simulink model "Group_20"  (R2024b)
settings: Solver=VariableStepAuto  StartTime=0.0  StopTime=inf  RelTol=1e-3
undefined symbols (not defined in the file or in its folder): Ion, Lithium
libraries: spsBatteryLib x3, spsIdealSwitchLib x3, spsSeriesRLCLoadLib x3, spsVoltageMeasurementLib x1, sps_lib x1
settings Model: Creator=om  LastModifiedBy=om

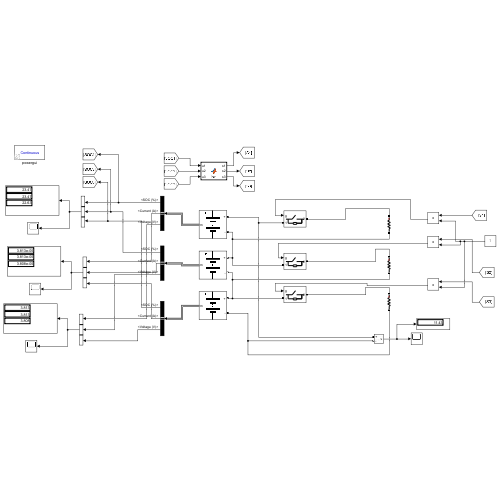
[thumbnail: Simulink's stored preview of the top-level diagram]
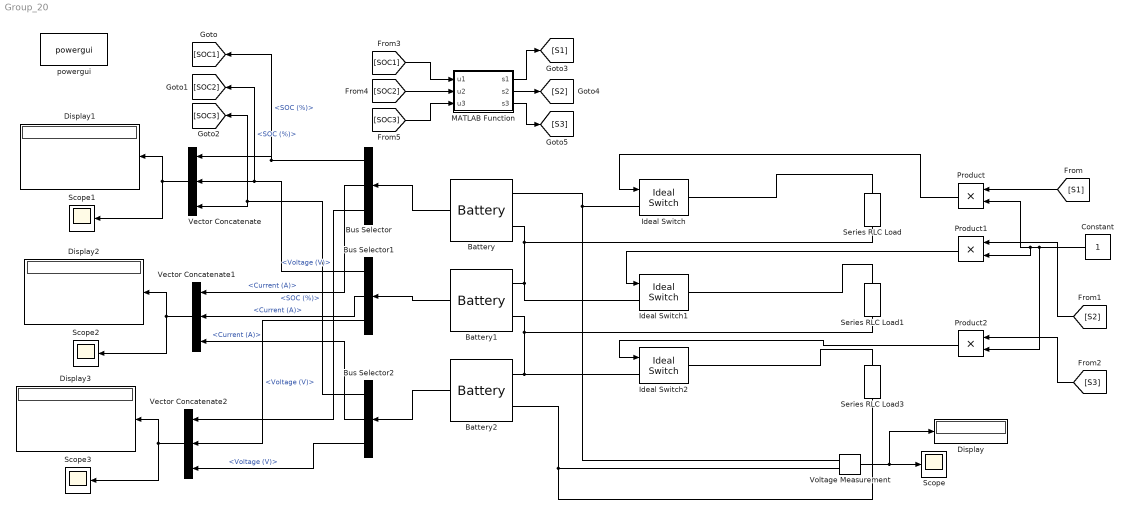
== system Group_20 ==
  Battery : spsBatteryLib/Battery  BatType=Lithium-Ion  NomV=3.6  NomQ=4.5  SOC=80  Batt_Tr=1  PresetModel=on  MaxQ=4.5  MinV=2.7  FullV=4.1904  Dis_rate=1.9565  R=0.008  Normal_OP=4.0696  expZone="[3.8894     0.22109]"
  Battery1 : spsBatteryLib/Battery  BatType=Lithium-Ion  NomV=3.6  NomQ=4.5  SOC=50  Batt_Tr=1  PresetModel=on  MaxQ=4.5  MinV=2.7  FullV=4.1904  Dis_rate=1.9565  R=0.008  Normal_OP=4.0696  expZone="[3.8894     0.22109]"
  Battery2 : spsBatteryLib/Battery  BatType=Lithium-Ion  NomV=3.6  NomQ=4.5  SOC=20  Batt_Tr=1  PresetModel=on  MaxQ=4.5  MinV=2.7  FullV=4.1904  Dis_rate=1.9565  R=0.008  Normal_OP=4.0696  expZone="[3.8894     0.22109]"
  Bus Selector : BusSelector  OutputSignals=SOC (%),Current (A),Voltage (V)
  Bus Selector1 : BusSelector  OutputSignals=SOC (%),Current (A),Voltage (V)
  Bus Selector2 : BusSelector  OutputSignals=SOC (%),Current (A),Voltage (V)
  Constant : Constant
  Display{,1..3} (4 alike) : Display
  Ideal Switch : spsIdealSwitchLib/Ideal Switch  Ron=0.001  Lon=0  IC=0  Rs=1e5  Cs=inf  Measurements=off
  Ideal Switch1 : spsIdealSwitchLib/Ideal Switch  Ron=0.001  Lon=0  IC=0  Rs=1e5  Cs=inf  Measurements=off
  Ideal Switch2 : spsIdealSwitchLib/Ideal Switch  Ron=0.001  Lon=0  IC=0  Rs=1e5  Cs=inf  Measurements=off
  MATLAB Function : MATLAB Function  TreatAsAtomicUnit=on
  Product : Product
  Product1 : Product
  Product2 : Product
  Scope{,1..3} (4 alike) : Scope
  Series RLC Load : spsSeriesRLCLoadLib/Series RLC Load  LConnTagsString=a  RConnTagsString=__new0  NominalVoltage=4  NominalFrequency=0.1  ActivePower=1000  InductivePower=0  CapacitivePower=0  Setx0=off  InitialVoltage=0  SetiL0=off  InitialCurrent=0  Measurements=None  LoadType=constant Z
  Series RLC Load1 : spsSeriesRLCLoadLib/Series RLC Load  LConnTagsString=a  RConnTagsString=__new0  NominalVoltage=4  NominalFrequency=0.1  ActivePower=1000  InductivePower=0  CapacitivePower=0  Setx0=off  InitialVoltage=0  SetiL0=off  InitialCurrent=0  Measurements=None  LoadType=constant Z
  Series RLC Load3 : spsSeriesRLCLoadLib/Series RLC Load  LConnTagsString=a  RConnTagsString=__new0  NominalVoltage=4  NominalFrequency=0.1  ActivePower=1000  InductivePower=0  CapacitivePower=0  Setx0=off  InitialVoltage=0  SetiL0=off  InitialCurrent=0  Measurements=None  LoadType=constant Z
  Vector Concatenate : Concatenate  NumInputs=3
  Vector Concatenate1 : Concatenate  NumInputs=3
  Vector Concatenate2 : Concatenate  NumInputs=3
  Voltage Measurement : spsVoltageMeasurementLib/Voltage Measurement  PhasorSimulation=off  OutputType=Complex  PSBequivalent=0
  powergui : sps_lib/powergui  Priority=1  SimulationMode=Continuous  SampleTime=50e-6  frequency=60  Iterations=50  frequencyindice=0  Pbase=100e6  ErrMax=1e-4  UnitsV=kV  UnitsW=MW  buscounter=0  FunctionMessages=off  echomessages=off  EnableUseOfTLC=off  CurrentSourceSwitches=off  DisableSnubberDevices=off  DisableRonSwitches=off  DisableVfSwitches=off  DisplayEquations=off  AutomaticDiscreteSolvers=off  SolverType=Tustin/Backward Euler (TBE)  Interpol=off  ExternalGateDelay=off  methode=off  Ts=100  x0status=blocks  SPID=on  SwTol=0  HookPort=off  NonlinearTolerance=1e-4  nMaxIteration=100  ContinueOnMaxIteration=off  RestoreLinks=warning  ResistiveCurrentMeasurement=off  Frange=[0:2:500]  Ylog=off  Xlog=on  ShowGrid=off  save=off  variable=ZData  structure=0  ZoomFFT=off  StartTime=0.0  cycles=1  DisplayStyle=1  fundamental=60  FreqAxis=off  MaxFrequency=1000  frequencyindicesteady=1  RmsSteady=1  display=off
  wires:
  Voltage Measurement/1 -> Display/1, Scope/1
  Product/1 -> Ideal Switch/1
  Product1/1 -> Ideal Switch1/1
  Product2/1 -> Ideal Switch2/1
  [S1] -> Product/1
  Constant/1 -> Product2/2, Product1/2, Product/2
  [S2] -> Product1/1
  [S3] -> Product2/1
  Battery/1 -> Bus Selector/1
  Battery2/1 -> Bus Selector2/1
  Battery1/1 -> Bus Selector1/1
  Vector Concatenate/1 -> Display1/1, Scope1/1
  Vector Concatenate1/1 -> Display2/1, Scope2/1
  Vector Concatenate2/1 -> Display3/1, Scope3/1
  Bus Selector/1 -> [SOC1], Vector Concatenate/1  "<SOC (%)>"
  Bus Selector1/1 -> [SOC2], Vector Concatenate/2  "<SOC (%)>"
  Bus Selector2/1 -> [SOC3], Vector Concatenate/3  "<SOC (%)>"
  Bus Selector/2 -> Vector Concatenate1/1  "<Current (A)>"
  Bus Selector1/2 -> Vector Concatenate1/2  "<Current (A)>"
  Bus Selector2/2 -> Vector Concatenate1/3  "<Current (A)>"
  Bus Selector/3 -> Vector Concatenate2/1  "<Voltage (V)>"
  Bus Selector1/3 -> Vector Concatenate2/2  "<Voltage (V)>"
  Bus Selector2/3 -> Vector Concatenate2/3  "<Voltage (V)>"
  [SOC1] -> MATLAB Function/1(u1)
  [SOC2] -> MATLAB Function/2(u2)
  [SOC3] -> MATLAB Function/3(u3)
  MATLAB Function/1(s1) -> [S1]
  MATLAB Function/2(s2) -> [S2]
  MATLAB Function/3(s3) -> [S3]
  connections:
  Battery/LConn2 -- Series RLC Load/RConn1 -- Ideal Switch1/LConn1 -- Battery1/LConn1
  Battery1/LConn2 -- Series RLC Load1/RConn1 -- Ideal Switch2/LConn1 -- Battery2/LConn1
  Ideal Switch/LConn1 -- Voltage Measurement/LConn1 -- Battery/LConn1
  Series RLC Load/LConn1 -- Ideal Switch/RConn1
  Series RLC Load1/LConn1 -- Ideal Switch1/RConn1
  Series RLC Load3/LConn1 -- Ideal Switch2/RConn1
  Series RLC Load3/RConn1 -- Battery2/LConn2 -- Voltage Measurement/LConn2

== matlab function Group_20/MATLAB Function ==
  data: u1 input; s1 output; s2 output; s3 output; u2 input; u3 input
function [s1,s2,s3] = fcn(u1,u2,u3)
u1=int32(u1)
u2=int32(u2)
u3=int32(u3)
if((u1>u2)||(u1>u3))
    s1=1;
else 
    s1=0;
end
if((u2>u1)||(u2>u3))
    s2=1;
else 
    s2=0;
end
if((u3>u1)||(u3>u2))
    s3=1;
else 
    s3=0;
end
